simulink model "TP1_Simulink_Con_Controlador_Mas_Perturbacion"  (R2021a)
settings: Solver=ode4  StartTime=0.0  StopTime=7000  FixedStep=0.1  RelTol=1e-3
values from neighbouring files (symbols this model uses):
  h0 = h0_vec(i)    [TP1.m]    (also in TP1_ParteMatlab.m = 0.45)
  Qi = 0.0001333    [TP1.m]    (also in TP1_ParteMatlab.m)
  u0 = Qi / (A_sal * sqrt(2 * g * h0))    [TP1.m]    (also in TP1_ParteMatlab.m)
libraries: cstblocks x3
settings Model: Creator=aghersin  LastModifiedBy=faust
settings SolverCC: AlgebraicLoopSolver=TrustRegion
settings DataIOCC: ReturnWorkspaceOutputs=off
settings OptimizationCC: LifeSpan=inf
settings DebuggingCC: SFExecutionAtInitializationDiag=none  SFMachineParentedDataDiag=warning  ArithmeticOperatorsInVariantConditions=warning
settings SFSimCC: SimUseLocalCustomCode=off  CustomCodeUndefinedFunction=UseInterfaceOnly
settings RTWCC: RTWUseLocalCustomCode=off
settings CodeAppCC: StateflowObjectComments=on

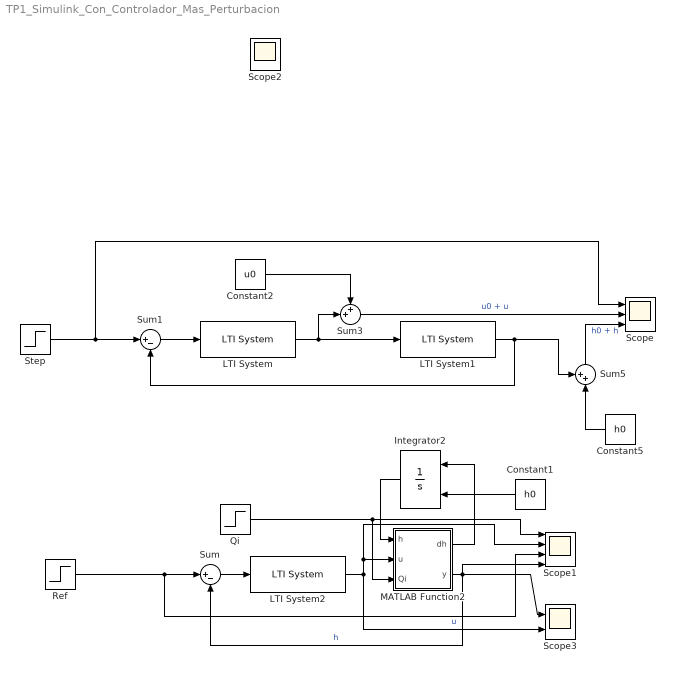
== system TP1_Simulink_Con_Controlador_Mas_Perturbacion ==
  Constant1 : Constant  Value=h0
  Constant2 : Constant  Value=u0
  Constant5 : Constant  Value=h0
  Integrator2 : Integrator  InitialConditionSource=external
  LTI System : cstblocks/LTI System  sys=C  IC=[]
  LTI System1 : cstblocks/LTI System  sys=P  IC=[]
  LTI System2 : cstblocks/LTI System  sys=C  IC=[]
  MATLAB Function2 : MATLAB Function  TreatAsAtomicUnit=on
  Qi : Step  Time=4700  Before=Qi  After=0.9 * Qi  SampleTime=0
  Ref : Step  Time=5000  Before=0.45  After=0.55  SampleTime=0
  Scope : Scope  NumInputPorts=3
  Scope1 : Scope  NumInputPorts=4
  Scope3 : Scope  NumInputPorts=2
  Step : Step  Time=3000  After=0.1  SampleTime=0
  Sum : Sum  Inputs=|+-
  Sum1 : Sum  Inputs=|+-
  Sum3 : Sum  Inputs=++|
  Sum5 : Sum  Inputs=++|
  Scope2 : Scope
  wires:
  Constant5/1 -> Sum5/2
  Step/1 -> Scope/1, Sum1/1
  Integrator2/1 -> MATLAB Function2/1(h)
  Constant1/1 -> Integrator2/2
  MATLAB Function2/2(y) -> Scope3/1, Sum/2, Scope1/4  "h"
  MATLAB Function2/1(dh) -> Integrator2/1
  Ref/1 -> Scope1/3, Sum/1
  LTI System2/1 -> Scope1/2, MATLAB Function2/2(u), Scope3/2  "u"
  Sum/1 -> LTI System2/1
  Sum1/1 -> LTI System/1
  LTI System1/1 -> Sum1/2, Sum5/1
  Constant2/1 -> Sum3/1
  LTI System/1 -> LTI System1/1, Sum3/2
  Sum3/1 -> Scope/2  "u0 + u"
  Sum5/1 -> Scope/3  "h0 + h"
  Qi/1 -> Scope1/1, MATLAB Function2/3(Qi)

== matlab function TP1_Simulink_Con_Controlador_Mas_Perturbacion/MATLAB Function2 ==
  data: h input; u input; dh output; y output; Qi input
function [dh,y] = fcn(h,u,Qi)
g = 9.8;        %En metros sobre segundo cuadrado
L = 0.9;        %En metros
L_h = 0.4;      %En metros
L_l = 0.1;      %En metros
d2 = 10.65e-3;
A_sal = pi * (d2 / 2)^2;
L1 = L_l /(L_h - L_l) * L;
dh = 3 * L1^2 * (Qi - A_sal * u * sqrt(2 * g * h))/(L_l^2 * (3 * h^2 + 6 * L1 * h + 3 * L1^2)) ;
y = h;
